simulink model "sxemJ"  (R2015b)
settings: Solver=VariableStepAuto  StartTime=0.0  StopTime=0.6  RelTol=1e-3
settings Model: Creator=hohotulca  LastModifiedBy=hohotulca

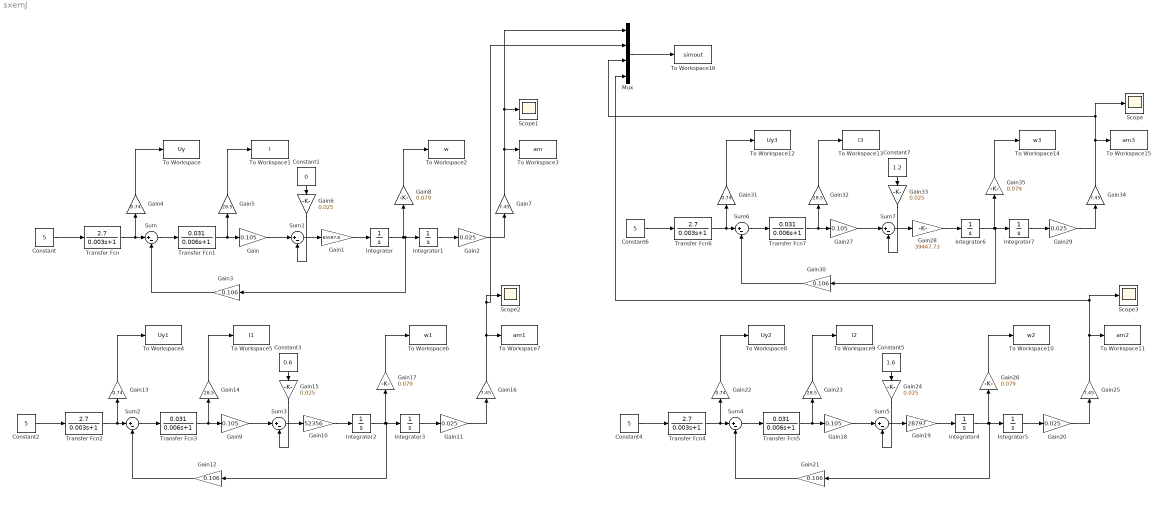
== system sxemJ ==
  Constant{,2,4,6} (4 alike) : Constant  Value=5
  Constant1 : Constant  Value=0
  Constant3 : Constant  Value=0.6
  Constant5 : Constant  Value=1.6
  Constant7 : Constant  Value=1.2
  Gain{,9,18,27} (4 alike) : Gain  Gain=0.105
  Gain1 : Gain  Gain=65597.8
  Gain10 : Gain  Gain=52356
  Gain{2,6,11,15,20,24,29,33} (8 alike) : Gain  Gain=0.025
  Gain{3,12,21,30} (4 alike) : Gain  Gain=0.106
  Gain{4,13,22,31} (4 alike) : Gain  Gain=0.74
  Gain{5,14,23,32} (4 alike) : Gain  Gain=28.5
  Gain{7,16,25,34} (4 alike) : Gain  Gain=7.45
  Gain{8,17,26,35} (4 alike) : Gain  Gain=0.079
  Gain19 : Gain  Gain=28797
  Gain28 : Gain  Gain=39447.73
  Integrator{,1..7} (8 alike) : Integrator
  Mux : Mux
  Scope{,1..3} (4 alike) : Scope
  Sum{,1..7} (8 alike) : Sum  Inputs=|+-
  To Workspace : ToWorkspace  VariableName=Uy  SaveFormat=Timeseries  SampleTime=-1
  To Workspace1 : ToWorkspace  VariableName=I  SaveFormat=Timeseries  SampleTime=-1
  To Workspace10 : ToWorkspace  VariableName=w2  SaveFormat=Timeseries  SampleTime=-1
  To Workspace11 : ToWorkspace  VariableName=am2  SaveFormat=Timeseries  SampleTime=-1
  To Workspace12 : ToWorkspace  VariableName=Uy3  SaveFormat=Timeseries  SampleTime=-1
  To Workspace13 : ToWorkspace  VariableName=I3  SaveFormat=Timeseries  SampleTime=-1
  To Workspace14 : ToWorkspace  VariableName=w3  SaveFormat=Timeseries  SampleTime=-1
  To Workspace15 : ToWorkspace  VariableName=am3  SaveFormat=Timeseries  SampleTime=-1
  To Workspace16 : ToWorkspace  VariableName=simout  SaveFormat=Timeseries  SampleTime=-1
  To Workspace2 : ToWorkspace  VariableName=w  SaveFormat=Timeseries  SampleTime=-1
  To Workspace3 : ToWorkspace  VariableName=am  SaveFormat=Timeseries  SampleTime=-1
  To Workspace4 : ToWorkspace  VariableName=Uy1  SaveFormat=Timeseries  SampleTime=-1
  To Workspace5 : ToWorkspace  VariableName=I1  SaveFormat=Timeseries  SampleTime=-1
  To Workspace6 : ToWorkspace  VariableName=w1  SaveFormat=Timeseries  SampleTime=-1
  To Workspace7 : ToWorkspace  VariableName=am1  SaveFormat=Timeseries  SampleTime=-1
  To Workspace8 : ToWorkspace  VariableName=Uy2  SaveFormat=Timeseries  SampleTime=-1
  To Workspace9 : ToWorkspace  VariableName=I2  SaveFormat=Timeseries  SampleTime=-1
  Transfer Fcn{,2,4,6} (4 alike) : TransferFcn  Numerator=[2.7]  Denominator=[0.003 1]
  Transfer Fcn{1,3,5,7} (4 alike) : TransferFcn  Numerator=[0.031]  Denominator=[0.006 1]
  wires:
  Constant/1 -> Transfer Fcn/1
  Transfer Fcn/1 -> Gain4/1, Sum/1
  Sum/1 -> Transfer Fcn1/1
  Transfer Fcn1/1 -> Gain5/1, Gain/1
  Gain/1 -> Sum1/1
  Sum1/1 -> Gain1/1
  Gain1/1 -> Integrator/1
  Integrator/1 -> Gain3/1, Integrator1/1, Gain8/1
  Integrator1/1 -> Gain2/1
  Gain3/1 -> Sum/2
  Gain4/1 -> To Workspace/1
  Gain5/1 -> To Workspace1/1
  Gain6/1 -> Sum1/2
  Constant1/1 -> Gain6/1
  Gain8/1 -> To Workspace2/1
  Gain7/1 -> Mux/1, Scope1/1, To Workspace3/1
  Gain2/1 -> Gain7/1
  Constant2/1 -> Transfer Fcn2/1
  Transfer Fcn2/1 -> Gain13/1, Sum2/1
  Sum2/1 -> Transfer Fcn3/1
  Transfer Fcn3/1 -> Gain14/1, Gain9/1
  Gain9/1 -> Sum3/1
  Sum3/1 -> Gain10/1
  Gain10/1 -> Integrator2/1
  Integrator2/1 -> Gain12/1, Integrator3/1, Gain17/1
  Integrator3/1 -> Gain11/1
  Gain12/1 -> Sum2/2
  Gain13/1 -> To Workspace4/1
  Gain14/1 -> To Workspace5/1
  Gain15/1 -> Sum3/2
  Constant3/1 -> Gain15/1
  Gain17/1 -> To Workspace6/1
  Gain11/1 -> Gain16/1
  Constant4/1 -> Transfer Fcn4/1
  Transfer Fcn4/1 -> Gain22/1, Sum4/1
  Sum4/1 -> Transfer Fcn5/1
  Transfer Fcn5/1 -> Gain23/1, Gain18/1
  Gain18/1 -> Sum5/1
  Sum5/1 -> Gain19/1
  Gain19/1 -> Integrator4/1
  Integrator4/1 -> Gain21/1, Integrator5/1, Gain26/1
  Integrator5/1 -> Gain20/1
  Gain21/1 -> Sum4/2
  Gain22/1 -> To Workspace8/1
  Gain23/1 -> To Workspace9/1
  Gain24/1 -> Sum5/2
  Constant5/1 -> Gain24/1
  Gain26/1 -> To Workspace10/1
  Gain25/1 -> Mux/4, Scope3/1, To Workspace11/1
  Gain20/1 -> Gain25/1
  Constant6/1 -> Transfer Fcn6/1
  Transfer Fcn6/1 -> Gain31/1, Sum6/1
  Sum6/1 -> Transfer Fcn7/1
  Transfer Fcn7/1 -> Gain32/1, Gain27/1
  Gain27/1 -> Sum7/1
  Sum7/1 -> Gain28/1
  Gain28/1 -> Integrator6/1
  Integrator6/1 -> Gain30/1, Integrator7/1, Gain35/1
  Integrator7/1 -> Gain29/1
  Gain30/1 -> Sum6/2
  Gain31/1 -> To Workspace12/1
  Gain32/1 -> To Workspace13/1
  Gain33/1 -> Sum7/2
  Constant7/1 -> Gain33/1
  Gain35/1 -> To Workspace14/1
  Gain34/1 -> Mux/3, Scope/1, To Workspace15/1
  Gain29/1 -> Gain34/1
  Mux/1 -> To Workspace16/1
  Gain16/1 -> Mux/2, Scope2/1, To Workspace7/1
